simulink model "Mod5Counter"  (R2020b)
settings: Solver=VariableStepAuto  StartTime=0.0  StopTime=10.0  RelTol=1e-3
settings Model: Creator=sayali  LastModifiedBy=sayali

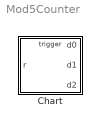
== system Mod5Counter ==
  Chart : Stateflow chart  TreatAsAtomicUnit=on

== stateflow chart Mod5Counter/Chart ==
  state digit0
    state zero
      en:
      d0=0;
    state one
      en:
      d0=1
    digit0.one -> digit0.zero [order 2] : [r==1]
    (default) -> digit0.zero
    digit0.one -> digit0.zero [order 1] : pulse{send(inc1);}
    digit0.zero -> digit0.one : pulse
  state digit1
    state zero
      en:
      d1=0;
    state one
      en:
      d1=1;
    (default) -> digit1.zero
    digit1.one -> digit1.zero : inc1{send(inc2);}
    digit1.zero -> digit1.one : inc1
  state digit2
    state zero
      en:
      d2=0;
    state one
      en:
      d2=1;
    (default) -> digit2.zero
    digit2.one -> digit2.zero : inc2
    digit2.zero -> digit2.one : inc2
  (default) -> digit0
  data: r input; d0 output; d1 output; d2 output
  events: pulse input RISING_EDGE_EVENT; inc1 local FUNCTION_CALL_EVENT; inc2 local FUNCTION_CALL_EVENT
